simulink model "VTOL_sim"  (R2017a)
settings: Solver=ode45  StartTime=0.0  StopTime=200  RelTol=1e-3  EnableMultiTasking=on
InitFcn:
  | param
undefined symbols (not defined in the file or in its folder): AP, diff_flat, drawVTOL, f_inv, grab_h, grab_output, grab_z, P, VTOL_ctrl
settings Model: Creator=beard  LastModifiedBy=jesse
settings DataIOCC: LimitDataPoints=on  SaveFormat=Array  SignalLoggingSaveFormat=ModelDataLogs
settings OptimizationCC: ExpressionDepthLimit=2147483647  InitFltsAndDblsToZero=on  LifeSpan=inf
settings DebuggingCC: UnderspecifiedInitializationDetection=Classic  MergeDetectMultiDrivingBlocksExec=none  SolverPrmCheckMsg=warning  FcnCallInpInsideContextMsg=warning  StateNameClashWarn=warning  SFUnexpectedBacktrackingDiag=warning  SFNoUnconditionalDefaultTransitionDiag=warning  SFExecutionAtInitializationDiag=none
settings HardwareCC: ProdBitPerPointer=32  ProdBitPerSizeT=32  ProdBitPerPtrDiffT=32  ProdLargestAtomicFloat=None  ProdIntDivRoundTo=Undefined  ProdEndianess=Unspecified  ProdWordSize=32  ProdHWDeviceType=32-bit Generic
settings ModelReferenceCC: PropagateSignalLabelsOutOfModel=off
settings GRTTargetCC: TargetLangStandard=C89/C90 (ANSI)  GeneratePreprocessorConditionals=Disable all  CombineOutputUpdateFcns=off  GRTInterface=on
settings ConfigComp: CovMetricSettings=dw  CovHtmlReporting=on  CovSaveCumulativeToWorkspaceVar=on  CovSaveSingleToWorkspaceVar=on  CovExternalEMLEnable=off

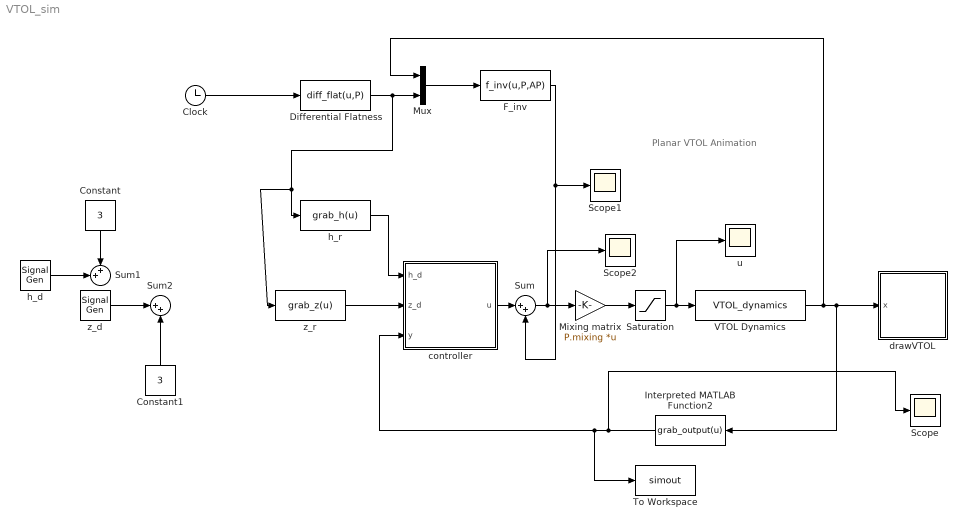
== system VTOL_sim ==
  note: Planar VTOL Animation
  Clock : Clock
  Constant : Constant  Value=3
  Constant1 : Constant  Value=3
  Differential Flatness : MATLABFcn  MATLABFcn=diff_flat(u,P)  OutputDimensions=6
  F_inv : MATLABFcn  MATLABFcn=f_inv(u,P,AP)  OutputDimensions=2
  Interpreted MATLAB Function2 : MATLABFcn  MATLABFcn=grab_output(u)  OutputDimensions=3
  Mixing matrix : Gain  Gain=P.mixing  Multiplication=Matrix(K*u)
  Mux : Mux  Inputs=2
  Saturation : Saturate  UpperLimit=P.fmax  LowerLimit=0
  Scope : Scope
  Scope1 : Scope
  Scope2 : Scope
  Sum : Sum  Inputs=|++
  Sum1 : Sum  Inputs=++|
  Sum2 : Sum  Inputs=|++
  To Workspace : ToWorkspace  VariableName=simout  SaveFormat=Timeseries  SampleTime=-1
  VTOL Dynamics : S-Function  FunctionName=VTOL_dynamics  Parameters=AP  SFunctionDeploymentMode=off  EnableBusSupport=off
  controller : Subsystem
  drawVTOL : Subsystem
      mask Display: image(imread('tv.jpg'))
  h_d : SignalGenerator  WaveForm=square  Amplitude=2.5  Frequency=.02
  h_r : MATLABFcn  MATLABFcn=grab_h(u)  OutputDimensions=1
  u : Scope
  z_d : SignalGenerator  WaveForm=square  Amplitude=2.5  Frequency=.008
  z_r : MATLABFcn  MATLABFcn=grab_z(u)  OutputDimensions=1
  wires:
  Constant/1 -> Sum1/1
  h_d/1 -> Sum1/2
  z_d/1 -> Sum2/1
  Constant1/1 -> Sum2/2
  Saturation/1 -> u/1, VTOL Dynamics/1
  Mixing matrix/1 -> Saturation/1
  Differential Flatness/1 -> z_r/1, h_r/1, Mux/2
  VTOL Dynamics/1 -> Mux/1, Interpreted MATLAB Function2/1, drawVTOL/1(x)
  Mux/1 -> F_inv/1
  Interpreted MATLAB Function2/1 -> Scope/1, To Workspace/1, controller/3(y)
  controller/1(u) -> Sum/1
  Sum/1 -> Scope2/1, Mixing matrix/1
  h_r/1 -> controller/1(h_d)
  z_r/1 -> controller/2(z_d)
  F_inv/1 -> Scope1/1, Sum/2
  Clock/1 -> Differential Flatness/1

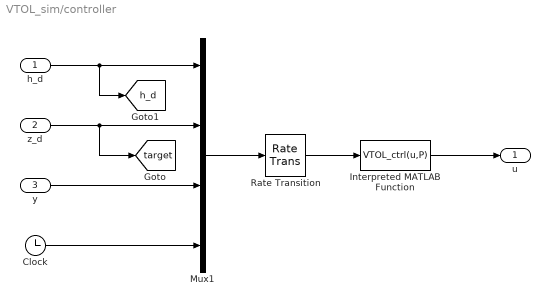
== system VTOL_sim/controller ==
  h_d : Inport
  z_d : Inport  Port=2
  y : Inport  Port=3
  Clock : Clock
  Interpreted MATLAB Function : MATLABFcn  MATLABFcn=VTOL_ctrl(u,P)  OutputDimensions=2
  Mux1 : Mux
  Rate Transition : RateTransition  OutPortSampleTime=P.Ts
  u : Outport
  tag scope: h_d=global, target=global
  wires:
  h_d/1 -> [h_d], Mux1/1
  Interpreted MATLAB Function/1 -> u/1
  Clock/1 -> Mux1/4
  y/1 -> Mux1/3
  z_d/1 -> [target], Mux1/2
  Mux1/1 -> Rate Transition/1
  Rate Transition/1 -> Interpreted MATLAB Function/1

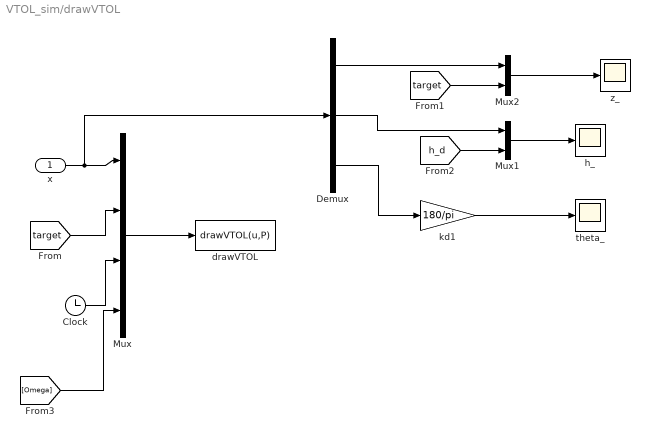
== system VTOL_sim/drawVTOL ==
  x : Inport
  Clock : Clock
  Demux : Demux  Outputs=3
  Mux : Mux
  Mux1 : Mux  Inputs=2
  Mux2 : Mux  Inputs=2
  drawVTOL : MATLABFcn  MATLABFcn=drawVTOL(u,P)  OutputDimensions=0  SampleTime=0.1
  h_ : Scope
  kd1 : Gain  Gain=180/pi
  theta_ : Scope
  z_ : Scope
  wires:
  Mux/1 -> drawVTOL/1
  x/1 -> Demux/1, Mux/1
  [target] -> Mux/2
  Mux1/1 -> h_/1
  Mux2/1 -> z_/1
  kd1/1 -> theta_/1
  Demux/3 -> kd1/1
  Demux/1 -> Mux2/1
  [target] -> Mux2/2
  Demux/2 -> Mux1/1
  [h_d] -> Mux1/2
  Clock/1 -> Mux/3
  [Omega] -> Mux/4
